simulink model "NeuromuscularModel2"  (R2019b)
settings: Solver=ode15s  StartTime=0.0  StopTime=20  MaxStep=.01  RelTol=1e-4  AbsTol=1e-6  EnableMultiTasking=on
values from neighbouring files (symbols this model uses):
  LceOffsetTA = 1-0.5*w    [ControlParams2.m]
  legLengthClr = .9    (= 0.9)    [ControlParams2.m]    (also in assignGains.m = Gains(20); assignGains2.m = Gains(20); assignGainsSagittal.m = GainsSagittal(39))
  LongDelay = 0.020    (= 0.02)    [ControlParams2.m]
  MidDelay = 0.010    (= 0.01)    [ControlParams2.m]
  N = 82    [vcmaes_1.5cm_0.9ms_Umb10_kneelim1_mstoptorque2.mat]
  ShortDelay = 0.005    [ControlParams2.m]
  simbiconGainD = 5*pi/180    (= 0.0872664625997)    [ControlParams2.m]    (also in assignGains.m = Gains(21); assignGains2.m = Gains(21); assignGainsSagittal.m = GainsSagittal(41))
  simbiconGainV = 5*pi/180    (= 0.0872664625997)    [ControlParams2.m]    (also in assignGains.m = Gains(22); assignGains2.m = Gains(22); assignGainsSagittal.m = GainsSagittal(42))
  simbiconLegAngle0 = 85*pi/180    (= 1.4835298642)    [ControlParams2.m]    (also in assignGains.m = Gains(23); assignGains2.m = Gains(23); assignGainsSagittal.m = GainsSagittal(40))
undefined symbols (not defined in the file or in its folder): footCenterToCGDist, footInertia, footMass, g, loptGAS, loptTA, lslackGAS, phimaxGASa, phimaxGASk, phirefGASa, phirefGASk, rGASa, rGASk, rhoGASa, rhoGASk, X, Y, Z
libraries: NeuroMuscularLibrary x89, nesl_utility x29, sm_lib x23, simulink x4, simulink_extras x2
(part 3 of 3)

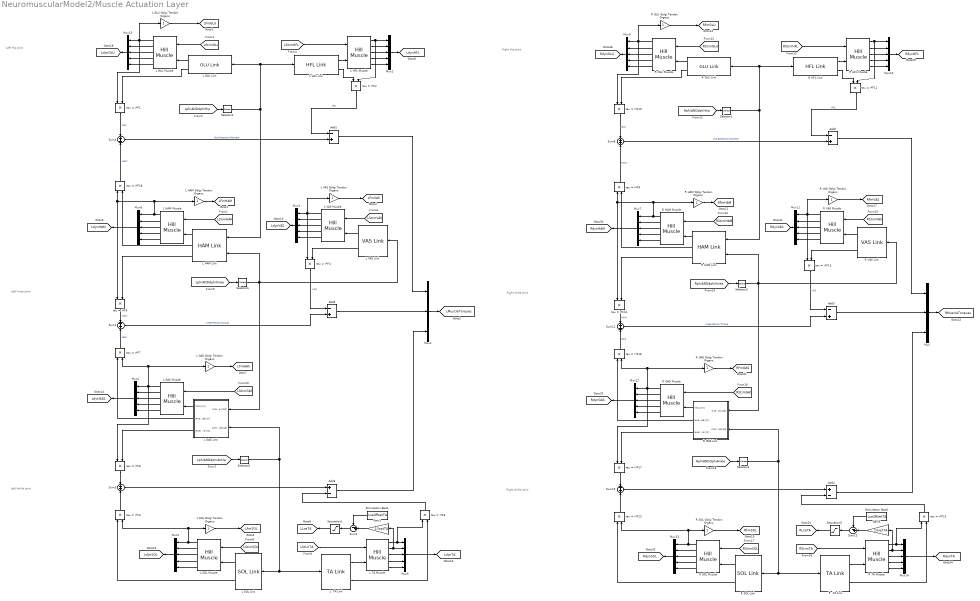
== system NeuromuscularModel2/Muscle Actuation Layer ==
  note: Right Hip Joint
  note: Right Knee Joint
  note: Right Ankle Joint
  note: Left Hip Joint
  note: Left Knee Joint
  note: Left Ankle Joint
  Add{1..3,5} (4 alike) : Sum  Inputs=-+
  Add4 : Sum  Inputs=+-
  Add6 : Sum  Inputs=+-
  Gain1 : Gain  Gain=1/loptTA
  Gain5 : Gain  Gain=1/loptTA
  L  TA Link : NeuroMuscularLibrary/TA Link  SystemSampleTime=-1  Latency=0  AutoFrameSizeCalculation=off
  L GAS Golgi Tendon Organs : Gain
  L GAS Link : Subsystem
  L GAS Muscle : NeuroMuscularLibrary/Hill Muscle  Fmax=FmaxGAS  lopt=loptGAS  vmax=vmaxGAS  lslack=lslackGAS
  L GLU Golgi Tendon Organs : Gain
  L GLU Link : NeuroMuscularLibrary/GLU Link  SystemSampleTime=-1  Latency=0  AutoFrameSizeCalculation=off
  L GLU Muscle : NeuroMuscularLibrary/Hill Muscle  Fmax=FmaxGLU  lopt=loptGLU  vmax=vmaxGLU  lslack=lslackGLU
  L HAM Golgi Tendon Organs : Gain
  L HAM Link : NeuroMuscularLibrary/HAM Link  SystemSampleTime=-1  Latency=0  AutoFrameSizeCalculation=off
  L HAM Muscle : NeuroMuscularLibrary/Hill Muscle  Fmax=FmaxHAM  lopt=loptHAM  vmax=vmaxHAM  lslack=lslackHAM
  L HFL Link : NeuroMuscularLibrary/HFL Link  SystemSampleTime=-1  Latency=0  AutoFrameSizeCalculation=off
  L HFL Muscle : NeuroMuscularLibrary/Hill Muscle  Fmax=FmaxHFL  lopt=loptHFL  vmax=vmaxHFL  lslack=lslackHFL
  L SOL Golgi Tendon Organs : Gain
  L SOL Link : NeuroMuscularLibrary/SOL Link  SystemSampleTime=-1  Latency=0  AutoFrameSizeCalculation=off
  L SOL Muscle : NeuroMuscularLibrary/Hill Muscle  Fmax=FmaxSOL  lopt=loptSOL  vmax=vmaxSOL  lslack=lslackSOL
  L TA Muscle : NeuroMuscularLibrary/Hill Muscle  Fmax=FmaxTA  lopt=loptTA  vmax=vmaxTA  lslack=lslackTA
  L VAS Golgi Tendon Organs : Gain
  L VAS Link : NeuroMuscularLibrary/VAS Link  SystemSampleTime=-1  Latency=0  AutoFrameSizeCalculation=off
  L VAS Muscle : NeuroMuscularLibrary/Hill Muscle  Fmax=FmaxVAS  lopt=loptVAS  vmax=vmaxVAS  lslack=lslackVAS
  Mux : Mux  Inputs=3
  Mux1 : Mux  Inputs=3
  Mux{2..15} (14 alike) : Mux  Inputs=5
  R  TA Link : NeuroMuscularLibrary/TA Link  SystemSampleTime=-1  Latency=0  AutoFrameSizeCalculation=off
  R GAS Golgi Tendon Organs : Gain
  R GAS Link : Subsystem
  R GAS Muscle : NeuroMuscularLibrary/Hill Muscle  Fmax=FmaxGAS  lopt=loptGAS  vmax=vmaxGAS  lslack=lslackGAS
  R GLU Golgi Tendon Organs : Gain
  R GLU Link : NeuroMuscularLibrary/GLU Link  SystemSampleTime=-1  Latency=0  AutoFrameSizeCalculation=off
  R GLU Muscle : NeuroMuscularLibrary/Hill Muscle  Fmax=FmaxGLU  lopt=loptGLU  vmax=vmaxGLU  lslack=lslackGLU
  R HAM Golgi Tendon Organs : Gain
  R HAM Link : NeuroMuscularLibrary/HAM Link  SystemSampleTime=-1  Latency=0  AutoFrameSizeCalculation=off
  R HAM Muscle : NeuroMuscularLibrary/Hill Muscle  Fmax=FmaxHAM  lopt=loptHAM  vmax=vmaxHAM  lslack=lslackHAM
  R HFL Link : NeuroMuscularLibrary/HFL Link  SystemSampleTime=-1  Latency=0  AutoFrameSizeCalculation=off
  R HFL Muscle : NeuroMuscularLibrary/Hill Muscle  Fmax=FmaxHFL  lopt=loptHFL  vmax=vmaxHFL  lslack=lslackHFL
  R SOL Golgi Tendon Organs : Gain
  R SOL Link : NeuroMuscularLibrary/SOL Link  SystemSampleTime=-1  Latency=0  AutoFrameSizeCalculation=off
  R SOL Muscle : NeuroMuscularLibrary/Hill Muscle  Fmax=FmaxSOL  lopt=loptSOL  vmax=vmaxSOL  lslack=lslackSOL
  R TA Muscle : NeuroMuscularLibrary/Hill Muscle  Fmax=FmaxTA  lopt=loptTA  vmax=vmaxTA  lslack=lslackTA
  R VAS Golgi Tendon Organs : Gain
  R VAS Link : NeuroMuscularLibrary/VAS Link  SystemSampleTime=-1  Latency=0  AutoFrameSizeCalculation=off
  R VAS Muscle : NeuroMuscularLibrary/Hill Muscle  Fmax=FmaxVAS  lopt=loptVAS  vmax=vmaxVAS  lslack=lslackVAS
  Saturation1 : Saturate  UpperLimit=inf  LowerLimit=0
  Saturation5 : Saturate  UpperLimit=inf  LowerLimit=0
  Selector{1..6} (6 alike) : Selector  InputPortWidth=2  IndexOptions=Index vector (dialog)  Indices=1  OutputSizes=1
  Stimulation Bias1 : Constant  Value=LceOffsetTA
  Stimulation Bias6 : Constant  Value=LceOffsetTA
  Sum{1,3..4,8,11,15} (6 alike) : Sum  Inputs=+|+
  Sum13 : Sum  Inputs=-+|
  Sum2 : Sum  Inputs=-+|
  tau = r*F{1..18} (18 alike) : Product
  tag scope: LFmGAS=global, LFmGLU=global, LFmHAM=global, LFmSOL=global, LFmVAS=global, LLceTA=global, LMuscleTorques=global, LdynGAS=global, LdynGLU=global, LdynHAM=global, LdynHFL=global, LdynSOL=global, LdynTA=global, LdynVAS=global, RFmGAS=global, RFmGLU=global, RFmHAM=global, RFmSOL=global, RFmVAS=global, RLceTA=global, RMuscleTorques=global, RdynGAS=global, RdynGLU=global, RdynHAM=global, RdynHFL=global, RdynSOL=global, RdynTA=global, RdynVAS=global
  wires:
  R HAM Link/1 -> R HAM Muscle/2
  R HAM Link/2 -> tau = r*F9/2
  R HAM Muscle/5 -> Mux7/5
  Mux7/1 -> [RdynHAM]
  R HAM Muscle/3 -> Mux7/3
  R HAM Muscle/4 -> Mux7/4
  [RphiANDdphiHip] -> Selector1/1
  Selector1/1 -> R HAM Link/1, R GLU Link/1, R HFL Link/1
  Add2/1 -> Mux/1
  R GLU Link/1 -> R GLU Muscle/2
  [RStimGLU] -> R GLU Muscle/1
  R GLU Muscle/5 -> Mux9/5
  R GLU Muscle/2 -> Mux9/2
  R GLU Muscle/3 -> Mux9/3
  R GLU Muscle/4 -> Mux9/4
  R GLU Link/2 -> tau = r*F10/2
  R GLU Muscle/1 -> Mux9/1, R GLU Golgi Tendon Organs/1, tau = r*F10/1
  R GLU Golgi Tendon Organs/1 -> [RFmGLU]
  R HFL Link/1 -> R HFL Muscle/2
  [RStimHFL] -> R HFL Muscle/1
  R HFL Muscle/2 -> Mux10/2
  R HFL Muscle/5 -> Mux10/5
  Mux10/1 -> [RdynHFL]
  R HFL Muscle/4 -> Mux10/4
  R HFL Muscle/3 -> Mux10/3
  R HFL Link/2 -> tau = r*F11/1
  R HFL Muscle/1 -> Mux10/1, tau = r*F11/2
  R HAM Muscle/2 -> Mux7/2
  R HAM Golgi Tendon Organs/1 -> [RFmHAM]
  [RStimHAM] -> R HAM Muscle/1
  Add3/1 -> Mux/2
  R VAS Link/1 -> R VAS Muscle/2
  R VAS Muscle/5 -> Mux11/5
  Mux11/1 -> [RdynVAS]
  R VAS Muscle/2 -> Mux11/2
  R VAS Muscle/3 -> Mux11/3
  R VAS Muscle/4 -> Mux11/4
  R VAS Muscle/1 -> R VAS Golgi Tendon Organs/1, Mux11/1, tau = r*F13/1
  R VAS Golgi Tendon Organs/1 -> [RFmVAS]
  R VAS Link/2 -> tau = r*F13/2
  R HAM Link/3 -> tau = r*F14/2
  Sum11/1 -> Add3/2  "Knee Flexion Torque"
  [RStimVAS] -> R VAS Muscle/1
  [RphiANDdphiKnee] -> Selector3/1
  R SOL Muscle/1 -> R SOL Golgi Tendon Organs/1, tau = r*F12/2, Mux13/1
  R SOL Muscle/5 -> Mux13/5
  Mux13/1 -> [RdynSOL]
  R SOL Muscle/2 -> Mux13/2
  R SOL Muscle/3 -> Mux13/3
  R SOL Muscle/4 -> Mux13/4
  R SOL Link/2 -> tau = r*F12/1
  R SOL Link/1 -> R SOL Muscle/2
  R SOL Golgi Tendon Organs/1 -> [RFmSOL]
  [RStimSOL] -> R SOL Muscle/1
  Selector2/1 -> R  TA Link/1, R SOL Link/1, R GAS Link/2(Ankle Angle[rad])
  [RphiANDdphiAnkle] -> Selector2/1
  Add4/1 -> Mux/3
  R  TA Link/1 -> R TA Muscle/2
  R TA Muscle/1 -> tau = r*F15/1, Mux14/1
  R TA Muscle/5 -> Mux14/5
  Mux14/1 -> [RdynTA]
  R TA Muscle/4 -> Mux14/4
  R TA Muscle/3 -> Mux14/3
  Sum13/1 -> Saturation5/1
  Saturation5/1 -> [RLceTA]
  [RStimTA] -> R TA Muscle/1
  Gain5/1 -> Sum13/2
  Stimulation Bias6/1 -> Sum13/1
  R  TA Link/2 -> tau = r*F15/2
  tau = r*F15/1 -> Add4/2
  R GAS Link/1(lmtu [m]) -> R GAS Muscle/2
  Selector3/1 -> R HAM Link/2, R VAS Link/1, R GAS Link/1(Knee Angle [rad])
  R GAS Muscle/5 -> Mux12/5
  Mux12/1 -> [RdynGAS]
  R GAS Muscle/2 -> Mux12/2
  R GAS Muscle/3 -> Mux12/3
  R GAS Muscle/4 -> Mux12/4
  R GAS Link/2(leverKnee [m]) -> tau = r*F16/1
  [RStimGAS] -> R GAS Muscle/1
  tau = r*F12/1 -> Sum15/2
  Sum15/1 -> Add4/1
  R GAS Link/3(leverAnkle [m]) -> tau = r*F17/2
  tau = r*F17/1 -> Sum15/1
  R GAS Muscle/1 -> Mux12/1, tau = r*F16/2, R GAS Golgi Tendon Organs/1, tau = r*F17/1
  R GAS Golgi Tendon Organs/1 -> [RFmGAS]
  tau = r*F9/1 -> Sum8/2  "HAM"
  tau = r*F10/1 -> Sum8/1  "GLU"
  tau = r*F11/1 -> Add2/1  "HFL"
  R HAM Muscle/1 -> tau = r*F14/1, tau = r*F9/1, R HAM Golgi Tendon Organs/1, Mux7/1
  Sum8/1 -> Add2/2  "Hip Extension Moment"
  tau = r*F16/1 -> Sum11/2  "GAS"
  tau = r*F14/1 -> Sum11/1  "HAM"
  tau = r*F13/1 -> Add3/1  "VAS"
  R TA Muscle/2 -> Gain5/1, Mux14/2
  Mux9/1 -> [RdynGLU]
  Mux/1 -> [RMuscleTorques]
  L HAM Link/1 -> L HAM Muscle/2
  L HAM Link/2 -> tau = r*F18/2
  L HAM Muscle/5 -> Mux8/5
  Mux8/1 -> [LdynHAM]
  L HAM Muscle/3 -> Mux8/3
  L HAM Muscle/4 -> Mux8/4
  [LphiANDdphiHip] -> Selector4/1
  Selector4/1 -> L HAM Link/1, L GLU Link/1, L HFL Link/1
  Add1/1 -> Mux1/1
  L GLU Link/1 -> L GLU Muscle/2
  [LStimGLU] -> L GLU Muscle/1
  L GLU Muscle/5 -> Mux15/5
  L GLU Muscle/2 -> Mux15/2
  L GLU Muscle/3 -> Mux15/3
  L GLU Muscle/4 -> Mux15/4
  L GLU Link/2 -> tau = r*F1/2
  L GLU Muscle/1 -> Mux15/1, L GLU Golgi Tendon Organs/1, tau = r*F1/1
  L GLU Golgi Tendon Organs/1 -> [LFmGLU]
  L HFL Link/1 -> L HFL Muscle/2
  [LStimHFL] -> L HFL Muscle/1
  L HFL Muscle/2 -> Mux2/2
  L HFL Muscle/5 -> Mux2/5
  Mux2/1 -> [LdynHFL]
  L HFL Muscle/4 -> Mux2/4
  L HFL Muscle/3 -> Mux2/3
  L HFL Link/2 -> tau = r*F2/1
  L HFL Muscle/1 -> Mux2/1, tau = r*F2/2
  L HAM Muscle/2 -> Mux8/2
  L HAM Golgi Tendon Organs/1 -> [LFmHAM]
  [LStimHAM] -> L HAM Muscle/1
  Add5/1 -> Mux1/2
  L VAS Link/1 -> L VAS Muscle/2
  L VAS Muscle/5 -> Mux3/5
  Mux3/1 -> [LdynVAS]
  L VAS Muscle/2 -> Mux3/2
  L VAS Muscle/3 -> Mux3/3
  L VAS Muscle/4 -> Mux3/4
  L VAS Muscle/1 -> L VAS Golgi Tendon Organs/1, Mux3/1, tau = r*F4/1
  L VAS Golgi Tendon Organs/1 -> [LFmVAS]
  L VAS Link/2 -> tau = r*F4/2
  L HAM Link/3 -> tau = r*F5/2
  Sum1/1 -> Add5/2  "Knee Flexion Torque"
  [LStimVAS] -> L VAS Muscle/1
  [LphiANDdphiKnee] -> Selector6/1
  L SOL Muscle/1 -> L SOL Golgi Tendon Organs/1, tau = r*F3/2, Mux5/1
  L SOL Muscle/5 -> Mux5/5
  Mux5/1 -> [LdynSOL]
  L SOL Muscle/2 -> Mux5/2
  L SOL Muscle/3 -> Mux5/3
  L SOL Muscle/4 -> Mux5/4
  L SOL Link/2 -> tau = r*F3/1
  L SOL Link/1 -> L SOL Muscle/2
  L SOL Golgi Tendon Organs/1 -> [LFmSOL]
  [LStimSOL] -> L SOL Muscle/1
  Selector5/1 -> L  TA Link/1, L SOL Link/1, L GAS Link/2(Ankle Angle[rad])
  [LphiANDdphiAnkle] -> Selector5/1
  Add6/1 -> Mux1/3
  L  TA Link/1 -> L TA Muscle/2
  L TA Muscle/1 -> tau = r*F6/1, Mux6/1
  L TA Muscle/5 -> Mux6/5
  Mux6/1 -> [LdynTA]
  L TA Muscle/4 -> Mux6/4
  L TA Muscle/3 -> Mux6/3
  Sum2/1 -> Saturation1/1
  Saturation1/1 -> [LLceTA]
  [LStimTA] -> L TA Muscle/1
  Gain1/1 -> Sum2/2
  Stimulation Bias1/1 -> Sum2/1
  L  TA Link/2 -> tau = r*F6/2
  tau = r*F6/1 -> Add6/2
  L GAS Link/1(lmtu [m]) -> L GAS Muscle/2
  Selector6/1 -> L HAM Link/2, L VAS Link/1, L GAS Link/1(Knee Angle [rad])
  L GAS Muscle/5 -> Mux4/5
  Mux4/1 -> [LdynGAS]
  L GAS Muscle/2 -> Mux4/2
  L GAS Muscle/3 -> Mux4/3
  L GAS Muscle/4 -> Mux4/4
  L GAS Link/2(leverKnee [m]) -> tau = r*F7/1
  [LStimGAS] -> L GAS Muscle/1
  tau = r*F3/1 -> Sum3/2
  Sum3/1 -> Add6/1
  L GAS Link/3(leverAnkle [m]) -> tau = r*F8/2
  tau = r*F8/1 -> Sum3/1
  L GAS Muscle/1 -> Mux4/1, tau = r*F7/2, L GAS Golgi Tendon Organs/1, tau = r*F8/1
  L GAS Golgi Tendon Organs/1 -> [LFmGAS]
  tau = r*F18/1 -> Sum4/2  "HAM"
  tau = r*F1/1 -> Sum4/1  "GLU"
  tau = r*F2/1 -> Add1/1  "HFL"
  L HAM Muscle/1 -> tau = r*F5/1, tau = r*F18/1, L HAM Golgi Tendon Organs/1, Mux8/1
  Sum4/1 -> Add1/2  "Hip Extension Moment"
  tau = r*F7/1 -> Sum1/2  "GAS"
  tau = r*F5/1 -> Sum1/1  "HAM"
  tau = r*F4/1 -> Add5/1  "VAS"
  L TA Muscle/2 -> Gain1/1, Mux6/2
  Mux15/1 -> [LdynGLU]
  Mux1/1 -> [LMuscleTorques]

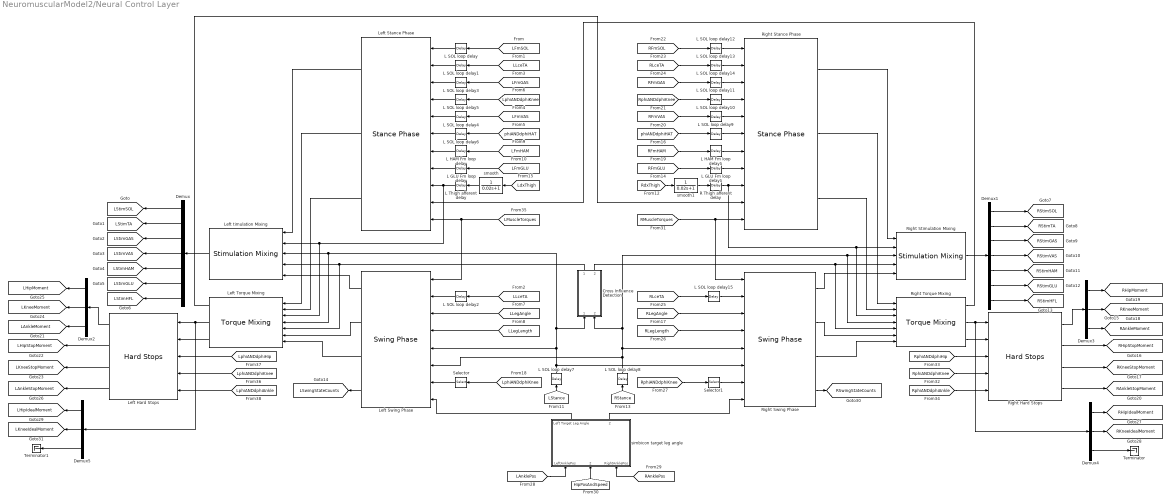
== system NeuromuscularModel2/Neural Control Layer ==
  Cross Influence Detection : Subsystem
  Demux : Demux  Outputs=7
  Demux1 : Demux  Outputs=7
  Demux{2..5} (4 alike) : Demux  Outputs=3
  L GLU Fm loop delay : TransportDelay  DelayTime=ShortDelay
  L GLU Fm loop delay1 : TransportDelay  DelayTime=ShortDelay
  L HAM Fm loop delay : TransportDelay  DelayTime=ShortDelay
  L HAM Fm loop delay1 : TransportDelay  DelayTime=ShortDelay
  L SOL loop delay{,1..3,12..15} (8 alike) : TransportDelay  DelayTime=LongDelay
  L SOL loop delay{4..5,7..8,10..11} (6 alike) : TransportDelay  DelayTime=MidDelay
  L SOL loop delay6 : TransportDelay  DelayTime=ShortDelay
  L SOL loop delay9 : TransportDelay  DelayTime=ShortDelay
  L Thigh afferent delay : TransportDelay  DelayTime=ShortDelay
  Left Hard Stops : NeuroMuscularLibrary/Hard Stops  SystemSampleTime=-1  Latency=0  AutoFrameSizeCalculation=off
  Left Stance Phase : NeuroMuscularLibrary/Stance Phase  GainHAM=GainHAM  GainGLU=GainGLU  GainSOL=GainSOL  GainSOLTA=GainSOLTA  GainTA=GainTA  GainGAS=GainGAS  GainVAS=GainVAS  GainKneeOverExt=GainKneeOverExt  PosGainGG=PosGainGG  SpeedGainGG=SpeedGainGG  Kglu=Kglu
  Left Swing Phase : NeuroMuscularLibrary/Swing Phase  GainTA=GainTA  hipPGain=hipPGain  hipDGain=hipDGain  legAngleFilter=legAngleFilter  kneeFlexGain=kneeFlexGain  kneeHoldGain1=kneeHoldGain1  kneeHoldGain2=kneeHoldGain2  kneeStopGain=kneeStopGain  kneeExtendGain=kneeExtendGain  legLengthClr=legLengthClr
  Left Torque Mixing : NeuroMuscularLibrary/Torque Mixing  SystemSampleTime=-1  Latency=0  AutoFrameSizeCalculation=off
  Left timulation Mixing : NeuroMuscularLibrary/Stimulation Mixing  SystemSampleTime=-1  Latency=0  AutoFrameSizeCalculation=off
  R Thigh afferent delay : TransportDelay  DelayTime=ShortDelay
  Right Hard Stops : NeuroMuscularLibrary/Hard Stops  SystemSampleTime=-1  Latency=0  AutoFrameSizeCalculation=off
  Right Stance Phase : NeuroMuscularLibrary/Stance Phase  GainHAM=GainHAM  GainGLU=GainGLU  GainSOL=GainSOL  GainSOLTA=GainSOLTA  GainTA=GainTA  GainGAS=GainGAS  GainVAS=GainVAS  GainKneeOverExt=GainKneeOverExt  PosGainGG=PosGainGG  SpeedGainGG=SpeedGainGG  Kglu=Kglu
  Right Stimulation Mixing : NeuroMuscularLibrary/Stimulation Mixing  SystemSampleTime=-1  Latency=0  AutoFrameSizeCalculation=off
  Right Swing Phase : NeuroMuscularLibrary/Swing Phase  GainTA=GainTA  hipPGain=hipPGain  hipDGain=hipDGain  legAngleFilter=legAngleFilter  kneeFlexGain=kneeFlexGain  kneeHoldGain1=kneeHoldGain1  kneeHoldGain2=kneeHoldGain2  kneeStopGain=kneeStopGain  kneeExtendGain=kneeExtendGain  legLengthClr=legLengthClr
  Right Torque Mixing : NeuroMuscularLibrary/Torque Mixing  SystemSampleTime=-1  Latency=0  AutoFrameSizeCalculation=off
  Selector : Selector  InputPortWidth=2  IndexOptions=Index vector (dialog)  Indices=2  OutputSizes=1
  Selector1 : Selector  InputPortWidth=2  IndexOptions=Index vector (dialog)  Indices=2  OutputSizes=1
  Terminator : Terminator
  Terminator1 : Terminator
  simbicon target leg angle : Subsystem
  smooth : TransferFcn  Denominator=[0.02 1]
  smooth1 : TransferFcn  Denominator=[0.02 1]
  tag scope: LAnkleMoment=global, LAnkleStopMoment=global, LHipIdealMoment=global, LHipMoment=global, LHipStopMoment=global, LKneeIdealMoment=global, LKneeMoment=global, LKneeStopMoment=global, LStimGAS=global, LStimGLU=global, LStimHAM=global, LStimHFL=global, LStimSOL=global, LStimTA=global, LStimVAS=global, LSwingStateCounts=global, RAnkleMoment=global, RAnkleStopMoment=global, RHipIdealMoment=global, RHipMoment=global, RHipStopMoment=global, RKneeIdealMoment=global, RKneeMoment=global, RKneeStopMoment=global, RStimGAS=global, RStimGLU=global, RStimHAM=global, RStimHFL=global, RStimSOL=global, RStimTA=global, RStimVAS=global, RSwingStateCounts=global
  wires:
  [LFmSOL] -> L SOL loop delay/1
  L SOL loop delay/1 -> Left Stance Phase/1
  [LLceTA] -> L SOL loop delay1/1
  L SOL loop delay1/1 -> Left Stance Phase/2
  Demux/1 -> [LStimSOL]
  Demux/2 -> [LStimTA]
  Demux/3 -> [LStimGAS]
  [LFmGAS] -> L SOL loop delay3/1
  L SOL loop delay3/1 -> Left Stance Phase/3
  [LLceTA] -> L SOL loop delay2/1
  L SOL loop delay4/1 -> Left Stance Phase/5
  [LFmVAS] -> L SOL loop delay4/1
  L SOL loop delay5/1 -> Left Stance Phase/4
  [LphiANDdphiKnee] -> L SOL loop delay5/1
  Demux/4 -> [LStimVAS]
  [phiANDdphiHAT] -> L SOL loop delay6/1
  L SOL loop delay6/1 -> Left Stance Phase/6
  Demux/5 -> [LStimHAM]
  Demux/6 -> [LStimGLU]
  Demux/7 -> [LStimHFL]
  [LdxThigh] -> smooth/1
  smooth/1 -> L Thigh afferent delay/1
  [RdxThigh] -> smooth1/1
  smooth1/1 -> R Thigh afferent delay/1
  [LFmHAM] -> L HAM Fm loop delay/1
  [LFmGLU] -> L GLU Fm loop delay/1
  L SOL loop delay7/1 -> Left Torque Mixing/4, Left timulation Mixing/3, Cross Influence Detection/1(LStance), Left Swing Phase/5, Right Swing Phase/6
  [RFmHAM] -> L HAM Fm loop delay1/1
  [RFmGLU] -> L GLU Fm loop delay1/1
  [phiANDdphiHAT] -> L SOL loop delay9/1
  L SOL loop delay9/1 -> Right Stance Phase/6
  Demux1/1 -> [RStimSOL]
  Demux1/2 -> [RStimTA]
  Demux1/4 -> [RStimVAS]
  Demux1/5 -> [RStimHAM]
  Demux1/7 -> [RStimHFL]
  Demux1/3 -> [RStimGAS]
  [LStance] -> L SOL loop delay7/1
  [RStance] -> L SOL loop delay8/1
  [RFmVAS] -> L SOL loop delay10/1
  [RphiANDdphiKnee] -> L SOL loop delay11/1
  L SOL loop delay10/1 -> Right Stance Phase/5
  L SOL loop delay11/1 -> Right Stance Phase/4
  L SOL loop delay12/1 -> Right Stance Phase/1
  [RFmSOL] -> L SOL loop delay12/1
  [RLceTA] -> L SOL loop delay13/1
  L SOL loop delay13/1 -> Right Stance Phase/2
  [RFmGAS] -> L SOL loop delay14/1
  L SOL loop delay14/1 -> Right Stance Phase/3
  [RLceTA] -> L SOL loop delay15/1
  Demux1/6 -> [RStimGLU]
  L Thigh afferent delay/1 -> Left Torque Mixing/3, Left timulation Mixing/2, Left Stance Phase/9
  L HAM Fm loop delay/1 -> Left Stance Phase/7
  L GLU Fm loop delay/1 -> Left Stance Phase/8
  R Thigh afferent delay/1 -> Right Stimulation Mixing/2, Right Torque Mixing/3, Right Stance Phase/9
  L HAM Fm loop delay1/1 -> Right Stance Phase/7
  L GLU Fm loop delay1/1 -> Right Stance Phase/8
  L SOL loop delay15/1 -> Right Swing Phase/2
  L SOL loop delay2/1 -> Left Swing Phase/2
  Right Stimulation Mixing/1 -> Demux1/1
  Right Stance Phase/1 -> Right Stimulation Mixing/1
  L SOL loop delay8/1 -> Right Stimulation Mixing/3, Right Torque Mixing/4, Cross Influence Detection/2(RStance), Right Swing Phase/5, Left Swing Phase/6
  Cross Influence Detection/2(LeftLeading) -> Right Stimulation Mixing/4, Right Torque Mixing/5
  Left timulation Mixing/1 -> Demux/1
  Left Stance Phase/1 -> Left timulation Mixing/1
  Cross Influence Detection/1(RightLeading) -> Left Torque Mixing/5, Left timulation Mixing/4
  Demux3/1 -> [RHipMoment]
  Demux3/2 -> [RKneeMoment]
  [LLegAngle] -> Left Swing Phase/3
  [LLegLength] -> Left Swing Phase/4
  [RLegAngle] -> Right Swing Phase/3
  [RLegLength] -> Right Swing Phase/4
  [RphiANDdphiKnee] -> Selector1/1
  Selector1/1 -> Right Swing Phase/7
  [LAnklePos] -> simbicon target leg angle/1(LeftAnklePos)
  [RAnklePos] -> simbicon target leg angle/3(RightAnklePos)
  Right Swing Phase/1 -> Right Stimulation Mixing/5
  [LphiANDdphiKnee] -> Selector/1
  Selector/1 -> Left Swing Phase/7
  Left Swing Phase/1 -> Left timulation Mixing/5
  [HipPosAndSpeed] -> simbicon target leg angle/2(HIPposAndSpeed)
  simbicon target leg angle/2(Right Target Leg Angle) -> Right Swing Phase/8
  simbicon target leg angle/1(Left Target Leg Angle) -> Left Swing Phase/8
  Right Swing Phase/4 -> [RSwingStateCounts]
  Left Swing Phase/4 -> [LSwingStateCounts]
  Demux3/3 -> [RAnkleMoment]
  [RphiANDdphiKnee] -> Right Hard Stops/4
  [RphiANDdphiHip] -> Right Hard Stops/3
  [RphiANDdphiAnkle] -> Right Hard Stops/5
  Right Hard Stops/2 -> [RHipStopMoment]
  Right Hard Stops/3 -> [RKneeStopMoment]
  Right Hard Stops/4 -> [RAnkleStopMoment]
  [LMuscleTorques] -> Left Swing Phase/1, Left Stance Phase/11
  Demux2/1 -> [LHipMoment]
  Demux2/3 -> [LAnkleMoment]
  Left Hard Stops/1 -> Demux2/1
  [LphiANDdphiKnee] -> Left Hard Stops/4
  [LphiANDdphiHip] -> Left Hard Stops/3
  Left Hard Stops/2 -> [LHipStopMoment]
  Left Hard Stops/3 -> [LKneeStopMoment]
  Left Hard Stops/4 -> [LAnkleStopMoment]
  Left Stance Phase/2 -> Left Torque Mixing/1
  Demux2/2 -> [LKneeMoment]
  Right Torque Mixing/2 -> Demux4/1, Right Hard Stops/1
  Right Hard Stops/1 -> Demux3/1
  [RMuscleTorques] -> Right Swing Phase/1, Right Stance Phase/11
  Demux4/1 -> [RHipIdealMoment]
  Demux4/2 -> [RKneeIdealMoment]
  Demux4/3 -> Terminator/1
  Right Swing Phase/3 -> Right Torque Mixing/7
  Right Swing Phase/2 -> Right Torque Mixing/6
  Right Stance Phase/3 -> Right Torque Mixing/2
  Right Stance Phase/2 -> Right Torque Mixing/1
  Right Torque Mixing/3 -> Right Hard Stops/2
  Right Torque Mixing/1 -> Left Stance Phase/10
  [LphiANDdphiAnkle] -> Left Hard Stops/5
  Left Torque Mixing/2 -> Demux5/1, Left Hard Stops/1
  Left Torque Mixing/3 -> Left Hard Stops/2
  Left Torque Mixing/1 -> Right Stance Phase/10
  Left Stance Phase/3 -> Left Torque Mixing/2
  Left Swing Phase/2 -> Left Torque Mixing/6
  Left Swing Phase/3 -> Left Torque Mixing/7
  Demux5/1 -> [LHipIdealMoment]
  Demux5/2 -> [LKneeIdealMoment]
  Demux5/3 -> Terminator1/1

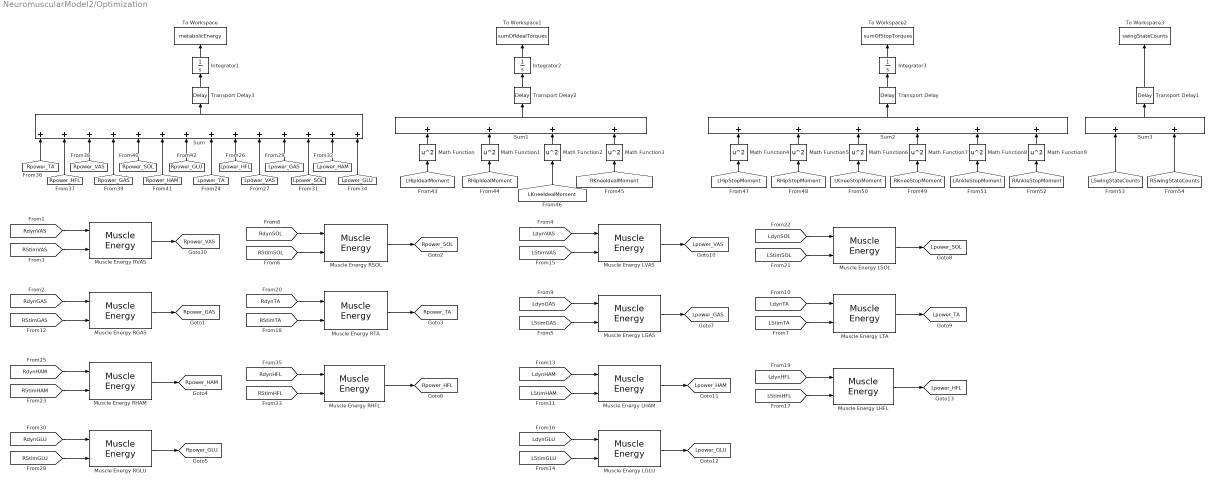
== system NeuromuscularModel2/Optimization ==
  Integrator1 : Integrator
  Integrator2 : Integrator
  Integrator3 : Integrator
  Math Function{,1..9} (10 alike) : Math  Operator=square  SaturateOnIntegerOverflow=on
  Muscle Energy LGAS : NeuroMuscularLibrary/Muscle Energy  lopt=loptGAS  FT=FT_GAS  Fmax=FmaxGAS
  Muscle Energy LGLU : NeuroMuscularLibrary/Muscle Energy  lopt=loptGLU  FT=FT_GLU  Fmax=FmaxGLU
  Muscle Energy LHAM : NeuroMuscularLibrary/Muscle Energy  lopt=loptHAM  FT=FT_HAM  Fmax=FmaxHAM
  Muscle Energy LHFL : NeuroMuscularLibrary/Muscle Energy  lopt=loptHFL  FT=FT_HFL  Fmax=FmaxHFL
  Muscle Energy LSOL : NeuroMuscularLibrary/Muscle Energy  lopt=loptSOL  FT=FT_SOL  Fmax=FmaxSOL
  Muscle Energy LTA : NeuroMuscularLibrary/Muscle Energy  lopt=loptTA  FT=FT_TA  Fmax=FmaxTA
  Muscle Energy LVAS : NeuroMuscularLibrary/Muscle Energy  lopt=loptVAS  FT=FT_VAS  Fmax=FmaxVAS
  Muscle Energy RGAS : NeuroMuscularLibrary/Muscle Energy  lopt=loptGAS  FT=FT_GAS  Fmax=FmaxGAS
  Muscle Energy RGLU : NeuroMuscularLibrary/Muscle Energy  lopt=loptGLU  FT=FT_GLU  Fmax=FmaxGLU
  Muscle Energy RHAM : NeuroMuscularLibrary/Muscle Energy  lopt=loptHAM  FT=FT_HAM  Fmax=FmaxHAM
  Muscle Energy RHFL : NeuroMuscularLibrary/Muscle Energy  lopt=loptHFL  FT=FT_HFL  Fmax=FmaxHFL
  Muscle Energy RSOL : NeuroMuscularLibrary/Muscle Energy  lopt=loptSOL  FT=FT_SOL  Fmax=FmaxSOL
  Muscle Energy RTA : NeuroMuscularLibrary/Muscle Energy  lopt=loptTA  FT=FT_TA  Fmax=FmaxTA
  Muscle Energy RVAS : NeuroMuscularLibrary/Muscle Energy  lopt=loptVAS  FT=FT_VAS  Fmax=FmaxVAS
  Sum : Sum  Inputs=++++++++++++++
  Sum1 : Sum  Inputs=++++
  Sum2 : Sum  Inputs=++++++
  Sum3 : Sum
  To Workspace : ToWorkspace  VariableName=metabolicEnergy  SampleTime=-1
      settings: MaxDataPoints=1
  To Workspace1 : ToWorkspace  VariableName=sumOfIdealTorques  SampleTime=-1
      settings: MaxDataPoints=1
  To Workspace2 : ToWorkspace  VariableName=sumOfStopTorques  SampleTime=-1
      settings: MaxDataPoints=1
  To Workspace3 : ToWorkspace  VariableName=swingStateCounts  SampleTime=-1
      settings: MaxDataPoints=1
  Transport Delay{,1..3} (4 alike) : TransportDelay  DelayTime=3  BufferSize=24576
  tag scope: Lpower_GAS=global, Lpower_GLU=global, Lpower_HAM=global, Lpower_HFL=global, Lpower_SOL=global, Lpower_TA=global, Lpower_VAS=global, Rpower_GAS=global, Rpower_GLU=global, Rpower_HAM=global, Rpower_HFL=global, Rpower_SOL=global, Rpower_TA=global, Rpower_VAS=global
  wires:
  [RdynSOL] -> Muscle Energy RSOL/1
  [RStimSOL] -> Muscle Energy RSOL/2
  [RStimVAS] -> Muscle Energy RVAS/2
  [RStimGAS] -> Muscle Energy RGAS/2
  Muscle Energy RVAS/1 -> [Rpower_VAS]
  Muscle Energy RGAS/1 -> [Rpower_GAS]
  Muscle Energy RSOL/1 -> [Rpower_SOL]
  Muscle Energy RTA/1 -> [Rpower_TA]
  [RdynTA] -> Muscle Energy RTA/1
  [RStimTA] -> Muscle Energy RTA/2
  [RdynHAM] -> Muscle Energy RHAM/1
  [RStimHAM] -> Muscle Energy RHAM/2
  [RdynGLU] -> Muscle Energy RGLU/1
  [RStimGLU] -> Muscle Energy RGLU/2
  [RdynHFL] -> Muscle Energy RHFL/1
  [RStimHFL] -> Muscle Energy RHFL/2
  Muscle Energy RHAM/1 -> [Rpower_HAM]
  Muscle Energy RGLU/1 -> [Rpower_GLU]
  Muscle Energy RHFL/1 -> [Rpower_HFL]
  [Rpower_TA] -> Sum/1
  [Rpower_GLU] -> Sum/7
  [Rpower_HAM] -> Sum/6
  [Rpower_SOL] -> Sum/5
  [Rpower_GAS] -> Sum/4
  [Rpower_VAS] -> Sum/3
  [Rpower_HFL] -> Sum/2
  [RdynGAS] -> Muscle Energy RGAS/1
  [RdynVAS] -> Muscle Energy RVAS/1
  [LdynSOL] -> Muscle Energy LSOL/1
  [LStimSOL] -> Muscle Energy LSOL/2
  [LStimVAS] -> Muscle Energy LVAS/2
  [LStimGAS] -> Muscle Energy LGAS/2
  Muscle Energy LVAS/1 -> [Lpower_VAS]
  Muscle Energy LGAS/1 -> [Lpower_GAS]
  Muscle Energy LSOL/1 -> [Lpower_SOL]
  Muscle Energy LTA/1 -> [Lpower_TA]
  [LdynTA] -> Muscle Energy LTA/1
  [LStimTA] -> Muscle Energy LTA/2
  [LdynHAM] -> Muscle Energy LHAM/1
  [LStimHAM] -> Muscle Energy LHAM/2
  [LdynGLU] -> Muscle Energy LGLU/1
  [LStimGLU] -> Muscle Energy LGLU/2
  [LdynHFL] -> Muscle Energy LHFL/1
  [LStimHFL] -> Muscle Energy LHFL/2
  Muscle Energy LHAM/1 -> [Lpower_HAM]
  Muscle Energy LGLU/1 -> [Lpower_GLU]
  Muscle Energy LHFL/1 -> [Lpower_HFL]
  [LdynGAS] -> Muscle Energy LGAS/1
  [LdynVAS] -> Muscle Energy LVAS/1
  [Lpower_TA] -> Sum/8
  [Lpower_GLU] -> Sum/14
  [Lpower_HAM] -> Sum/13
  [Lpower_SOL] -> Sum/12
  [Lpower_GAS] -> Sum/11
  [Lpower_VAS] -> Sum/10
  [Lpower_HFL] -> Sum/9
  Integrator1/1 -> To Workspace/1
  Sum/1 -> Transport Delay3/1
  Integrator2/1 -> To Workspace1/1
  Sum1/1 -> Transport Delay2/1
  Math Function/1 -> Sum1/1
  [LHipIdealMoment] -> Math Function/1
  Math Function1/1 -> Sum1/2
  [RHipIdealMoment] -> Math Function1/1
  Math Function2/1 -> Sum1/3
  Math Function3/1 -> Sum1/4
  [LKneeIdealMoment] -> Math Function2/1
  [RKneeIdealMoment] -> Math Function3/1
  Integrator3/1 -> To Workspace2/1
  Math Function4/1 -> Sum2/1
  [LHipStopMoment] -> Math Function4/1
  Math Function5/1 -> Sum2/2
  [RHipStopMoment] -> Math Function5/1
  Math Function6/1 -> Sum2/3
  Math Function7/1 -> Sum2/4
  [LKneeStopMoment] -> Math Function6/1
  [RKneeStopMoment] -> Math Function7/1
  [LAnkleStopMoment] -> Math Function8/1
  Math Function8/1 -> Sum2/5
  [RAnkleStopMoment] -> Math Function9/1
  Math Function9/1 -> Sum2/6
  Transport Delay/1 -> Integrator3/1
  Sum2/1 -> Transport Delay/1
  Sum3/1 -> Transport Delay1/1
  Transport Delay1/1 -> To Workspace3/1
  [LSwingStateCounts] -> Sum3/1
  [RSwingStateCounts] -> Sum3/2
  Transport Delay2/1 -> Integrator2/1
  Transport Delay3/1 -> Integrator1/1

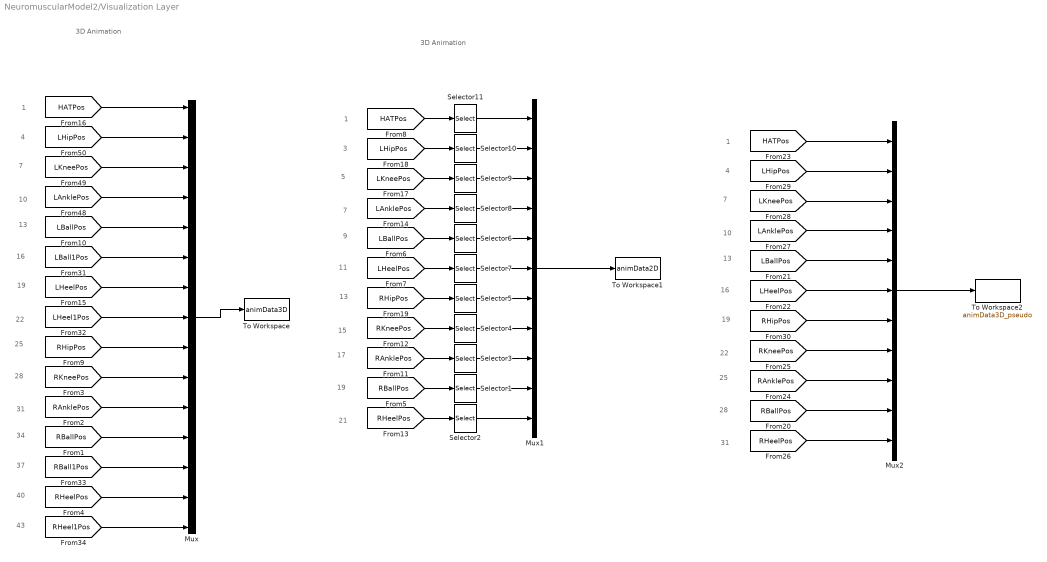
== system NeuromuscularModel2/Visualization Layer ==
  note: 31
  note: 28
  note: 25
  note: 22
  note: 19
  note: 16
  note: 13
  note: 10
  note: 7
  note: 4
  note: 1
  note: 3D Animation
  note: 21
  note: 17
  note: 11
  note: 7
  note: 15
  note: 9
  note: 3
  note: 1
  note: 13
  note: 3D Animation
  note: 19
  note: 5
  note: 28
  note: 22
  note: 19
  note: 16
  note: 10
  note: 7
  note: 1
  note: 4
  note: 13
  note: 31
  note: 25
  note: 34
  note: 37
  note: 40
  note: 43
  Mux : Mux  Inputs=15
  Mux1 : Mux  Inputs=11
  Mux2 : Mux  Inputs=11
  Selector{1..11} (11 alike) : Selector  InputPortWidth=3  IndexOptions=Index vector (dialog)  Indices=[1 3]  OutputSizes=1
  To Workspace : ToWorkspace  VariableName=animData3D  SaveFormat=Structure With Time  SampleTime=1/30
  To Workspace1 : ToWorkspace  VariableName=animData2D  SaveFormat=Structure With Time  SampleTime=1/30
  To Workspace2 : ToWorkspace  VariableName=animData3D_pseudo  SaveFormat=Structure With Time  SampleTime=1/30
  wires:
  [HATPos] -> Mux/1
  [LBallPos] -> Mux/5
  [LAnklePos] -> Mux/4
  [LKneePos] -> Mux/3
  [LHipPos] -> Mux/2
  Mux/1 -> To Workspace/1
  [LHeelPos] -> Selector7/1
  Selector3/1 -> Mux1/9
  Selector1/1 -> Mux1/10
  Selector6/1 -> Mux1/5
  Selector2/1 -> Mux1/11
  [LKneePos] -> Selector9/1
  Selector5/1 -> Mux1/7
  Selector4/1 -> Mux1/8
  [LAnklePos] -> Selector8/1
  Selector8/1 -> Mux1/4
  Selector9/1 -> Mux1/3
  [LHipPos] -> Selector10/1
  Selector7/1 -> Mux1/6
  [LBallPos] -> Selector6/1
  Selector10/1 -> Mux1/2
  [HATPos] -> Selector11/1
  [RHipPos] -> Selector5/1
  [RHeelPos] -> Selector2/1
  [RAnklePos] -> Selector3/1
  Mux1/1 -> To Workspace1/1
  [RBallPos] -> Selector1/1
  [RKneePos] -> Selector4/1
  Selector11/1 -> Mux1/1
  [RKneePos] -> Mux2/8
  [RHipPos] -> Mux2/7
  Mux2/1 -> To Workspace2/1
  [RAnklePos] -> Mux2/9
  [LAnklePos] -> Mux2/4
  [LHipPos] -> Mux2/2
  [LHeelPos] -> Mux2/6
  [LKneePos] -> Mux2/3
  [RHeelPos] -> Mux2/11
  [HATPos] -> Mux2/1
  [LBallPos] -> Mux2/5
  [RBallPos] -> Mux2/10
  [LBall1Pos] -> Mux/6
  [LHeelPos] -> Mux/7
  [LHeel1Pos] -> Mux/8
  [RHipPos] -> Mux/9
  [RKneePos] -> Mux/10
  [RAnklePos] -> Mux/11
  [RBallPos] -> Mux/12
  [RBall1Pos] -> Mux/13
  [RHeelPos] -> Mux/14
  [RHeel1Pos] -> Mux/15

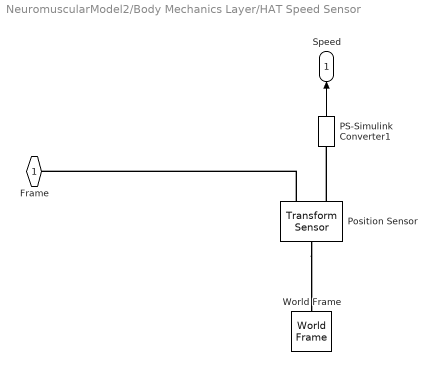
== system NeuromuscularModel2/Body Mechanics Layer/HAT Speed Sensor ==
  PS-Simulink Converter1 : nesl_utility/PS-Simulink Converter  PhysicalDomain=network_engine_domain  SubClassName=ps_output  LeftPortType=input  RightPortType=output  PseudoPeriodic=off  Frequencies=[]  Unit=m/s  AffineConversion=off
  Position Sensor : sm_lib/Frames and Transforms/Transform Sensor  MeasurementFrame=World  SenseAngle=off  SenseAxis=off  SenseAngle1=off  SenseAngle2=off  SenseAngle3=off  SenseQ=off  SenseR=off  SenseOmegaX=off  SenseOmegaY=off  SenseOmegaZ=off  SenseOmega1=off  SenseOmega2=off  SenseOmega3=off  SenseQDot=off  SenseRDot=off  SenseAlphaX=off  SenseAlphaY=off  SenseAlphaZ=off  SenseAlpha1=off  SenseAlpha2=off  SenseAlpha3=off  SenseQDDot=off  SenseRDDot=off  SenseX=off  SenseY=off  SenseZ=off  SenseRad=off  SenseAzim=off  SenseDist=off  SenseInc=off  SenseXDot=on  SenseYDot=off  SenseZDot=off  SenseRadDot=off  SenseAzimDot=off  SenseDistDot=off  SenseIncDot=off  SenseXDDot=off  SenseYDDot=off  SenseZDDot=off  SenseRadDDot=off  SenseAzimDDot=off  SenseDistDDot=off  SenseIncDDot=off
  World Frame : sm_lib/Frames and Transforms/World Frame
  Frame : PMIOPort  Side=Left
  Speed : Outport
  wires:
  PS-Simulink Converter1/1 -> Speed/1
  connections:
  Position Sensor/LConn1 -- World Frame/RConn1
  Position Sensor/RConn1 -- Frame/RConn1
  Position Sensor/RConn2 -- PS-Simulink Converter1/LConn1

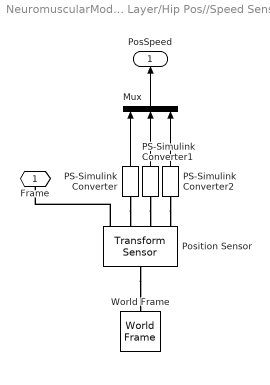
== system NeuromuscularModel2/Body Mechanics Layer/Hip Pos//Speed Sensor ==
  Mux : Mux  Inputs=3
  PS-Simulink Converter : nesl_utility/PS-Simulink Converter  PhysicalDomain=network_engine_domain  SubClassName=ps_output  LeftPortType=input  RightPortType=output  PseudoPeriodic=off  Frequencies=[]  Unit=m  AffineConversion=off
  PS-Simulink Converter1 : nesl_utility/PS-Simulink Converter  PhysicalDomain=network_engine_domain  SubClassName=ps_output  LeftPortType=input  RightPortType=output  PseudoPeriodic=off  Frequencies=[]  Unit=m  AffineConversion=off
  PS-Simulink Converter2 : nesl_utility/PS-Simulink Converter  PhysicalDomain=network_engine_domain  SubClassName=ps_output  LeftPortType=input  RightPortType=output  PseudoPeriodic=off  Frequencies=[]  Unit=m/s  AffineConversion=off
  Position Sensor : sm_lib/Frames and Transforms/Transform Sensor  MeasurementFrame=World  SenseAngle=off  SenseAxis=off  SenseAngle1=off  SenseAngle2=off  SenseAngle3=off  SenseQ=off  SenseR=off  SenseOmegaX=off  SenseOmegaY=off  SenseOmegaZ=off  SenseOmega1=off  SenseOmega2=off  SenseOmega3=off  SenseQDot=off  SenseRDot=off  SenseAlphaX=off  SenseAlphaY=off  SenseAlphaZ=off  SenseAlpha1=off  SenseAlpha2=off  SenseAlpha3=off  SenseQDDot=off  SenseRDDot=off  SenseX=on  SenseY=off  SenseZ=on  SenseRad=off  SenseAzim=off  SenseDist=off  SenseInc=off  SenseXDot=on  SenseYDot=off  SenseZDot=off  SenseRadDot=off  SenseAzimDot=off  SenseDistDot=off  SenseIncDot=off  SenseXDDot=off  SenseYDDot=off  SenseZDDot=off  SenseRadDDot=off  SenseAzimDDot=off  SenseDistDDot=off  SenseIncDDot=off
  World Frame : sm_lib/Frames and Transforms/World Frame
  Frame : PMIOPort  Side=Left
  PosSpeed : Outport
  wires:
  Mux/1 -> PosSpeed/1
  PS-Simulink Converter/1 -> Mux/1
  PS-Simulink Converter1/1 -> Mux/2
  PS-Simulink Converter2/1 -> Mux/3
  connections:
  Position Sensor/LConn1 -- World Frame/RConn1
  Position Sensor/RConn1 -- Frame/RConn1
  PS-Simulink Converter/LConn1 -- Position Sensor/RConn2
  PS-Simulink Converter1/LConn1 -- Position Sensor/RConn3
  PS-Simulink Converter2/LConn1 -- Position Sensor/RConn4

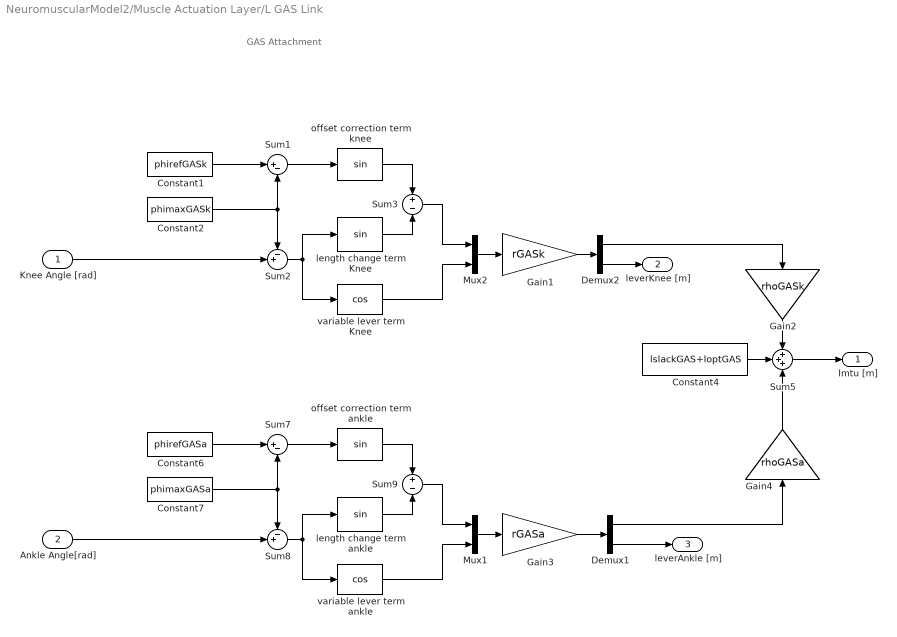
== system NeuromuscularModel2/Muscle Actuation Layer/L GAS Link ==
  note: GAS Attachment
  Knee Angle [rad] : Inport
  Ankle Angle[rad] : Inport  Port=2
  Constant1 : Constant  Value=phirefGASk
  Constant2 : Constant  Value=phimaxGASk
  Constant4 : Constant  Value=lslackGAS+loptGAS
  Constant6 : Constant  Value=phirefGASa
  Constant7 : Constant  Value=phimaxGASa
  Demux1 : Demux  Outputs=2
  Demux2 : Demux  Outputs=2
  Gain1 : Gain  Gain=rGASk
  Gain2 : Gain  Gain=rhoGASk
  Gain3 : Gain  Gain=rGASa
  Gain4 : Gain  Gain=rhoGASa
  Mux1 : Mux  Inputs=2
  Mux2 : Mux  Inputs=2
  Sum1 : Sum  Inputs=|+-
  Sum2 : Sum  Inputs=-+|
  Sum3 : Sum  Inputs=+-
  Sum5 : Sum  Inputs=+++
  Sum7 : Sum  Inputs=|+-
  Sum8 : Sum  Inputs=-+|
  Sum9 : Sum  Inputs=+-
  length change term Knee : Trigonometry
  length change term ankle : Trigonometry
  offset correction term ankle : Trigonometry
  offset correction term knee : Trigonometry
  variable lever term Knee : Trigonometry  Operator=cos
  variable lever term ankle : Trigonometry  Operator=cos
  lmtu [m] : Outport
  leverKnee [m] : Outport  Port=2
  leverAnkle [m] : Outport  Port=3
  wires:
  Ankle Angle[rad]/1 -> Sum8/2
  Sum5/1 -> lmtu [m]/1
  variable lever term ankle/1 -> Mux1/2
  Demux1/2 -> leverAnkle [m]/1
  Sum8/1 -> variable lever term ankle/1, length change term ankle/1
  Constant7/1 -> Sum8/1, Sum7/2
  Sum7/1 -> offset correction term ankle/1
  Constant6/1 -> Sum7/1
  length change term ankle/1 -> Sum9/2
  offset correction term ankle/1 -> Sum9/1
  Sum9/1 -> Mux1/1
  Constant4/1 -> Sum5/2
  Mux1/1 -> Gain3/1
  Gain3/1 -> Demux1/1
  Demux1/1 -> Gain4/1
  Gain4/1 -> Sum5/3
  Knee Angle [rad]/1 -> Sum2/2
  variable lever term Knee/1 -> Mux2/2
  Sum2/1 -> variable lever term Knee/1, length change term Knee/1
  Constant2/1 -> Sum2/1, Sum1/2
  Sum1/1 -> offset correction term knee/1
  Constant1/1 -> Sum1/1
  length change term Knee/1 -> Sum3/2
  offset correction term knee/1 -> Sum3/1
  Sum3/1 -> Mux2/1
  Mux2/1 -> Gain1/1
  Gain1/1 -> Demux2/1
  Demux2/2 -> leverKnee [m]/1
  Demux2/1 -> Gain2/1
  Gain2/1 -> Sum5/1

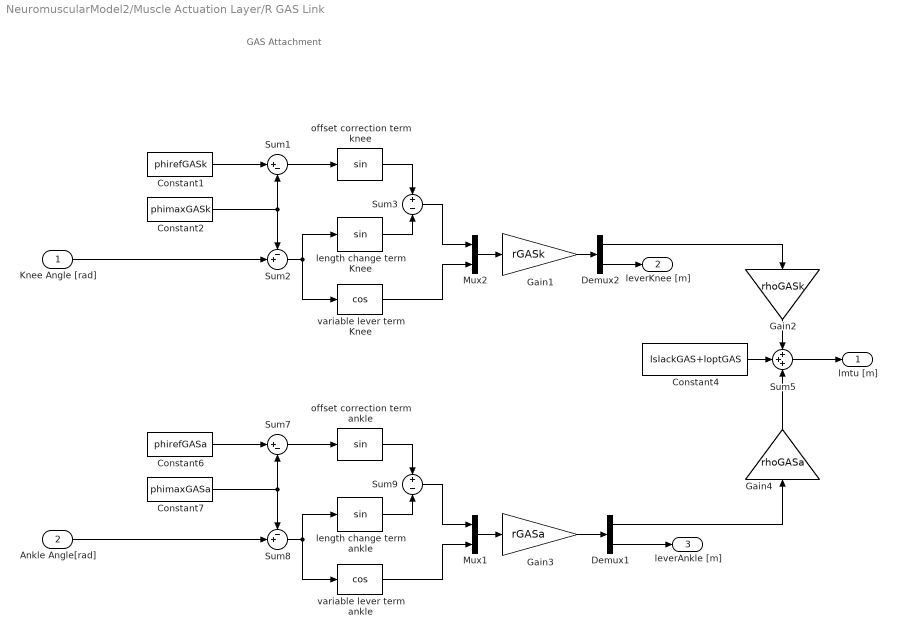
== system NeuromuscularModel2/Muscle Actuation Layer/R GAS Link ==
  note: GAS Attachment
  Knee Angle [rad] : Inport
  Ankle Angle[rad] : Inport  Port=2
  Constant1 : Constant  Value=phirefGASk
  Constant2 : Constant  Value=phimaxGASk
  Constant4 : Constant  Value=lslackGAS+loptGAS
  Constant6 : Constant  Value=phirefGASa
  Constant7 : Constant  Value=phimaxGASa
  Demux1 : Demux  Outputs=2
  Demux2 : Demux  Outputs=2
  Gain1 : Gain  Gain=rGASk
  Gain2 : Gain  Gain=rhoGASk
  Gain3 : Gain  Gain=rGASa
  Gain4 : Gain  Gain=rhoGASa
  Mux1 : Mux  Inputs=2
  Mux2 : Mux  Inputs=2
  Sum1 : Sum  Inputs=|+-
  Sum2 : Sum  Inputs=-+|
  Sum3 : Sum  Inputs=+-
  Sum5 : Sum  Inputs=+++
  Sum7 : Sum  Inputs=|+-
  Sum8 : Sum  Inputs=-+|
  Sum9 : Sum  Inputs=+-
  length change term Knee : Trigonometry
  length change term ankle : Trigonometry
  offset correction term ankle : Trigonometry
  offset correction term knee : Trigonometry
  variable lever term Knee : Trigonometry  Operator=cos
  variable lever term ankle : Trigonometry  Operator=cos
  lmtu [m] : Outport
  leverKnee [m] : Outport  Port=2
  leverAnkle [m] : Outport  Port=3
  wires:
  Ankle Angle[rad]/1 -> Sum8/2
  Sum5/1 -> lmtu [m]/1
  variable lever term ankle/1 -> Mux1/2
  Demux1/2 -> leverAnkle [m]/1
  Sum8/1 -> variable lever term ankle/1, length change term ankle/1
  Constant7/1 -> Sum8/1, Sum7/2
  Sum7/1 -> offset correction term ankle/1
  Constant6/1 -> Sum7/1
  length change term ankle/1 -> Sum9/2
  offset correction term ankle/1 -> Sum9/1
  Sum9/1 -> Mux1/1
  Constant4/1 -> Sum5/2
  Mux1/1 -> Gain3/1
  Gain3/1 -> Demux1/1
  Demux1/1 -> Gain4/1
  Gain4/1 -> Sum5/3
  Knee Angle [rad]/1 -> Sum2/2
  variable lever term Knee/1 -> Mux2/2
  Sum2/1 -> variable lever term Knee/1, length change term Knee/1
  Constant2/1 -> Sum2/1, Sum1/2
  Sum1/1 -> offset correction term knee/1
  Constant1/1 -> Sum1/1
  length change term Knee/1 -> Sum3/2
  offset correction term knee/1 -> Sum3/1
  Sum3/1 -> Mux2/1
  Mux2/1 -> Gain1/1
  Gain1/1 -> Demux2/1
  Demux2/2 -> leverKnee [m]/1
  Demux2/1 -> Gain2/1
  Gain2/1 -> Sum5/1

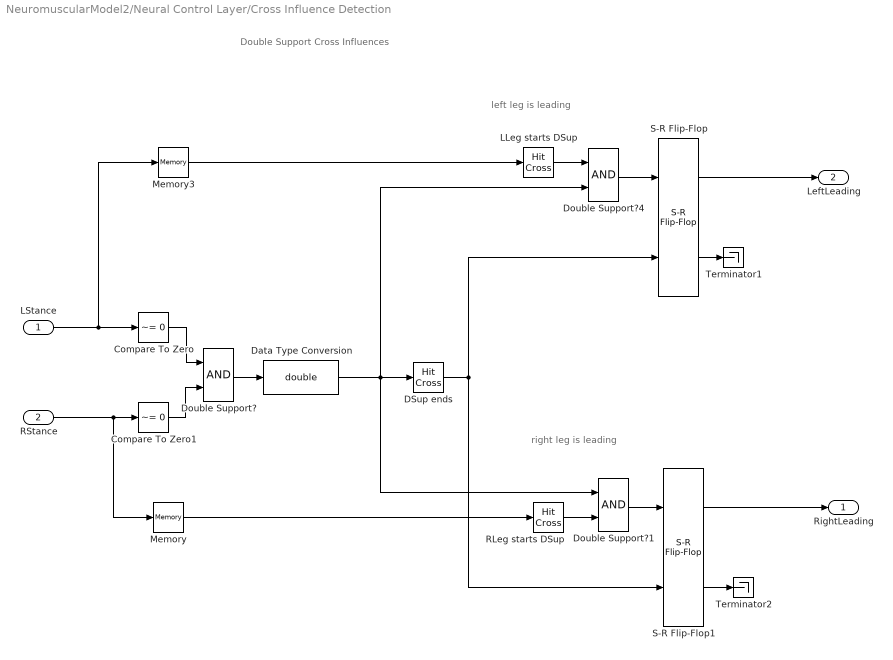
== system NeuromuscularModel2/Neural Control Layer/Cross Influence Detection ==
  note: right leg is leading
  note: left leg is leading
  note: Double Support Cross Influences
  LStance : Inport
  RStance : Inport  Port=2
  Compare To Zero : simulink/Logic and Bit Operations/Compare To Zero  relop=~=  OutDataTypeStr=boolean
  Compare To Zero1 : simulink/Logic and Bit Operations/Compare To Zero  relop=~=  OutDataTypeStr=boolean
  DSup ends : HitCross  HitCrossingOffset=0.5  HitCrossingDirection=falling  ZeroCross=off
  Data Type Conversion : DataTypeConversion  OutDataTypeStr=double
  Double Support? : Logic  AllPortsSameDT=off
  Double Support?1 : Logic  AllPortsSameDT=off
  Double Support?4 : Logic  AllPortsSameDT=off
  LLeg starts DSup : HitCross  HitCrossingOffset=0.5  HitCrossingDirection=rising  ZeroCross=off
  Memory : Memory
  Memory3 : Memory
  RLeg starts DSup : HitCross  HitCrossingOffset=0.5  HitCrossingDirection=rising  ZeroCross=off
  S-R Flip-Flop : simulink_extras/Flip Flops/S-R Flip-Flop  initial_condition=0
  S-R Flip-Flop1 : simulink_extras/Flip Flops/S-R Flip-Flop  initial_condition=0
  Terminator1 : Terminator
  Terminator2 : Terminator
  RightLeading : Outport
  LeftLeading : Outport  Port=2
  wires:
  S-R Flip-Flop/2 -> Terminator1/1
  S-R Flip-Flop/1 -> LeftLeading/1
  S-R Flip-Flop1/2 -> Terminator2/1
  LStance/1 -> Memory3/1, Compare To Zero/1
  RStance/1 -> Compare To Zero1/1, Memory/1
  S-R Flip-Flop1/1 -> RightLeading/1
  Memory/1 -> RLeg starts DSup/1
  RLeg starts DSup/1 -> Double Support?1/2
  Double Support?1/1 -> S-R Flip-Flop1/1
  Memory3/1 -> LLeg starts DSup/1
  LLeg starts DSup/1 -> Double Support?4/1
  Double Support?4/1 -> S-R Flip-Flop/1
  DSup ends/1 -> S-R Flip-Flop/2, S-R Flip-Flop1/2
  Compare To Zero/1 -> Double Support?/1
  Compare To Zero1/1 -> Double Support?/2
  Double Support?/1 -> Data Type Conversion/1
  Data Type Conversion/1 -> Double Support?1/1, Double Support?4/2, DSup ends/1

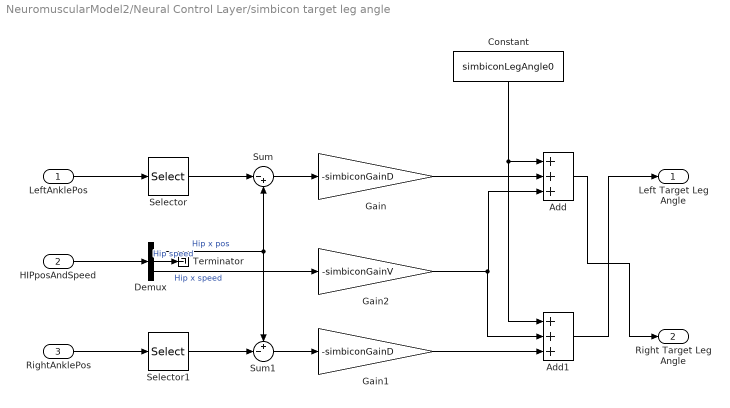
== system NeuromuscularModel2/Neural Control Layer/simbicon target leg angle ==
  LeftAnklePos : Inport
  HIPposAndSpeed : Inport  Port=2
  RightAnklePos : Inport  Port=3
  Add : Sum  Inputs=+++
  Add1 : Sum  Inputs=+++
  Constant : Constant  Value=simbiconLegAngle0
  Demux : Demux  Outputs=3
  Gain : Gain  Gain=-simbiconGainD
  Gain1 : Gain  Gain=-simbiconGainD
  Gain2 : Gain  Gain=-simbiconGainV
  Selector : Selector  InputPortWidth=3  IndexOptions=Index vector (dialog)  Indices=[1]  OutputSizes=1
  Selector1 : Selector  InputPortWidth=3  IndexOptions=Index vector (dialog)  Indices=[1]  OutputSizes=1
  Sum : Sum  Inputs=|-+
  Sum1 : Sum  Inputs=+-|
  Terminator : Terminator
  Left Target Leg Angle : Outport
  Right Target Leg Angle : Outport  Port=2
  wires:
  HIPposAndSpeed/1 -> Demux/1
  Demux/1 -> Sum/2, Sum1/1  "Hip x pos"
  Sum/1 -> Gain/1
  Sum1/1 -> Gain1/1
  Gain/1 -> Add/2
  Gain2/1 -> Add1/2, Add/3
  Gain1/1 -> Add1/3
  Constant/1 -> Add/1, Add1/1
  Add1/1 -> Left Target Leg Angle/1
  Add/1 -> Right Target Leg Angle/1
  LeftAnklePos/1 -> Selector/1
  Selector/1 -> Sum/1
  RightAnklePos/1 -> Selector1/1
  Selector1/1 -> Sum1/2
  Demux/3 -> Gain2/1  "Hip x speed"
  Demux/2 -> Terminator/1  "Hip speed"
